simulink library "lib_transmission"  (Simulink 4.1.1)
undefined symbols (not defined in the file or in its folder): fc_map_spd, fc_max_trq, fc_spd_scale, fc_trq_scale, fd_inertia, fd_loss, fd_ratio, gb_inertia, gb_loss_const, gb_loss_input_spd_coeff, gb_loss_input_trq_coeff, gb_loss_output_spd_coeff, gb_loss_output_trq_coeff, gb_map_spd_out, gb_map_trq_in, gb_map_trq_out, gb_ratio, gb_spd_scale, gb_trq_scale, htc_inertia, htc_k_adv, htc_k_adv_coast, htc_max_coast_tr, htc_min_coast_tr, htc_sr, htc_sr_coast, htc_tr, htc_tr_coast, mc_map_spd, mc_max_trq, mc_overtrq_factor, mc_spd_scale, mc_trq_scale, tc_loss, tc_mc_to_fc_ratio, tx_eff_map, tx_map_spd, tx_map_trq, tx_pg_r, tx_pg_s, vc_idle_spd, vc_launch_spd
libraries: lib_transmission x2
(part 2 of 3)

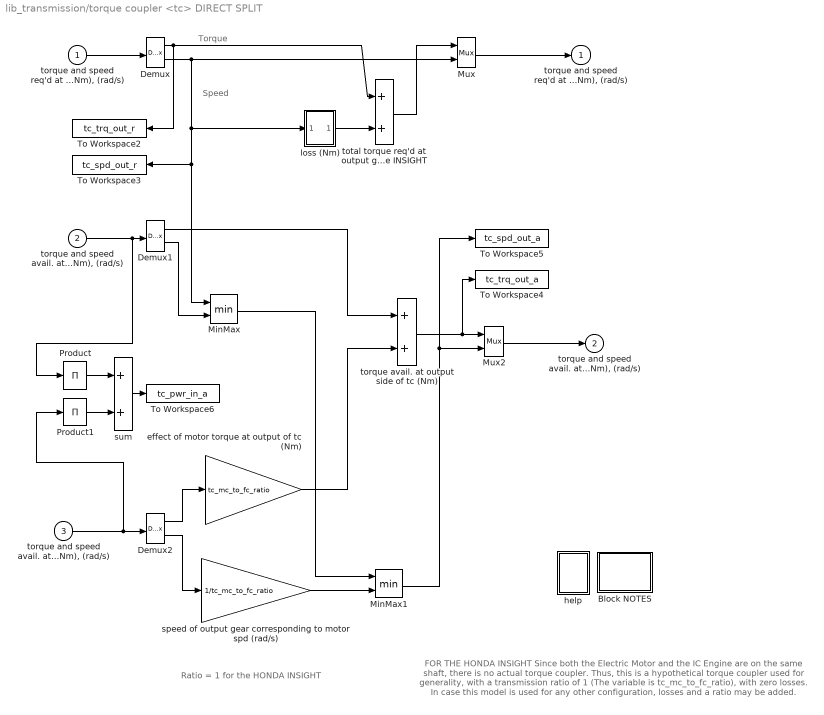
== system lib_transmission/torque coupler <tc> DIRECT SPLIT ==
  note: FOR THE HONDA INSIGHT
      | Since both the Electric Motor and the IC Engine are on the same shaft,
      | there is no actual torque coupler. Thus, this is a hypothetical torque coupler used for
      | generality, with a transmission ratio of 1 (The variable is tc_mc_to_fc_ratio),
      | with zero losses. In case this model is used for any other configuration, losses
      | and a ratio may be added.
  note: Ratio = 1 for the HONDA INSIGHT
  note: Torque
  note: Speed
  "torque and speed req'd at output side of torque coupler (Nm), (rad/s)" : Inport  Port=1  LatchInput=off
  "torque and speed avail. at main input (Nm), (rad/s)" : Inport  Port=2  LatchInput=off
  "torque and speed avail. at motor input to tc (Nm), (rad/s)" : Inport  Port=3  LatchInput=off
  Block NOTES : Subsystem
      settings: RTWFcnNameOpts=Auto  RTWFileNameOpts=Auto
      mask Display: disp('Block\nNOTES')
  Demux : Demux  Outputs=2  BusSelectionMode=off
  Demux1 : Demux  Outputs=2  BusSelectionMode=off
  Demux2 : Demux  Outputs=2  BusSelectionMode=off
  MinMax : MinMax  Function=min  Inputs=2
  MinMax1 : MinMax  Function=min  Inputs=2
  Mux : Mux  Inputs=2
      settings: DisplayOption=none
  Mux2 : Mux  Inputs=2
      settings: DisplayOption=none
  Product : Product  Inputs=1  Multiplication=Element-wise(.*)  SaturateOnIntegerOverflow=on
  Product1 : Product  Inputs=1  Multiplication=Element-wise(.*)  SaturateOnIntegerOverflow=on
  To Workspace2 : ToWorkspace  VariableName=tc_trq_out_r  SampleTime=-1  SaveFormat=Array
  To Workspace3 : ToWorkspace  VariableName=tc_spd_out_r  SampleTime=-1  SaveFormat=Array
  To Workspace4 : ToWorkspace  VariableName=tc_trq_out_a  SampleTime=-1  SaveFormat=Array
  To Workspace5 : ToWorkspace  VariableName=tc_spd_out_a  SampleTime=-1  SaveFormat=Array
  To Workspace6 : ToWorkspace  VariableName=tc_pwr_in_a  SampleTime=-1  SaveFormat=Array
  effect of motor torque at output of tc (Nm) : Gain  Gain=tc_mc_to_fc_ratio  Multiplication=Element-wise(K.*u)  SaturateOnIntegerOverflow=on
  help : Subsystem
      settings: OpenFcn=web(['file:\\\' which('torque_coupler.htm')]);  RTWFcnNameOpts=Auto  RTWFileNameOpts=Auto
      mask Display: image(imread('doc_man.jpg'))
  loss (Nm) : Subsystem
      settings: RTWFcnNameOpts=Auto  RTWFileNameOpts=Auto
  speed of output gear corresponding to motor spd (rad/s) : Gain  Gain=1/tc_mc_to_fc_ratio  Multiplication=Element-wise(K.*u)  SaturateOnIntegerOverflow=on
  "sum " : Sum  Inputs=++  SaturateOnIntegerOverflow=on
  torque avail. at output side of tc (Nm) : Sum  Inputs=++  SaturateOnIntegerOverflow=on
  total torque req'd at output gear (Nm) Loss==0 for the INSIGHT : Sum  Inputs=++  SaturateOnIntegerOverflow=on
  "torque and speed req'd at main input to torque coupler (Nm), (rad/s)" : Outport  Port=1  InitialOutput=0
  "torque and speed avail. at output side of torque coupler (Nm), (rad/s)" : Outport  Port=2  InitialOutput=0
  wires:
  MinMax1/1 -> To Workspace5/1, Mux2/2
  speed of output gear corresponding to motor spd (rad/s)/1 -> MinMax1/2
  Demux2/2 -> speed of output gear corresponding to motor spd (rad/s)/1
  effect of motor torque at output of tc (Nm)/1 -> torque avail. at output side of tc (Nm)/2
  Demux2/1 -> effect of motor torque at output of tc (Nm)/1
  Demux1/2 -> MinMax/2
  "torque and speed req'd at output side of torque coupler (Nm), (rad/s)"/1 -> Demux/1
  Mux/1 -> "torque and speed req'd at main input to torque coupler (Nm), (rad/s)"/1
  "sum "/1 -> To Workspace6/1
  Product/1 -> "sum "/1
  "torque and speed avail. at main input (Nm), (rad/s)"/1 -> Demux1/1, Product/1
  "torque and speed avail. at motor input to tc (Nm), (rad/s)"/1 -> Demux2/1, Product1/1
  Product1/1 -> "sum "/2
  Demux1/1 -> torque avail. at output side of tc (Nm)/1
  MinMax/1 -> MinMax1/1
  Mux2/1 -> "torque and speed avail. at output side of torque coupler (Nm), (rad/s)"/1
  torque avail. at output side of tc (Nm)/1 -> To Workspace4/1, Mux2/1
  Demux/2 -> To Workspace3/1, MinMax/1, loss (Nm)/1(tc output speed (rad/s)), Mux/2
  Demux/1 -> To Workspace2/1, total torque req'd at output gear (Nm) Loss==0 for the INSIGHT/1
  loss (Nm)/1(drag torque (Nm)) -> total torque req'd at output gear (Nm) Loss==0 for the INSIGHT/2
  total torque req'd at output gear (Nm) Loss==0 for the INSIGHT/1 -> Mux/1

== system lib_transmission/CVT gearbox  <gb>/Block NOTES1 ==
  note: This gearbox model includes loss data, rotational inertia, and a gear reduction.
  note: The loss torque is zero when the gears are not turning,
      | and is applied at the input side of the gear reduction.
  note: The inertia torque is the input torque required to accelerate the
      | final drive's inertia as measured on the input side.
  note: Available output torque is estimated assuming that the gearbox efficiency for theavailable input
      | torque andspeed is the same as the gearbox efficiency for the REQUESTED input torque.
  note: This is a good assumption, at least for the VW 4-speed manual transaxle of SAE 820741.
      | In the VW transaxle, efficiency is fairly independent of torque and speed at high torques.

== system lib_transmission/CVT gearbox  <gb>/Pout/Pin, neglecting inertia ==
  note: Pout/Pin, neglecting inertia, is used to estimate the output torque given the
      | input torque in a very simple forward-facing calculation.
  Tin : Inport  Port=1  LatchInput=off
  Tinertia : Inport  Port=2  LatchInput=off
  Tout : Inport  Port=3  LatchInput=off
  gear ratio : Inport  Port=4  LatchInput=off
  Constant : Constant  Orientation=up  Value=eps
  Constant2 : Constant  Orientation=left  Value=0.5
  Pout/Pin (neglecting inertia) : Product  Inputs=*/  Multiplication=Element-wise(.*)  SaturateOnIntegerOverflow=on
  Product : Product  Inputs=2  Multiplication=Element-wise(.*)  SaturateOnIntegerOverflow=on
  Switch : Switch  Threshold=eps
  Tin-Tinertia : Sum  Inputs=+-  SaturateOnIntegerOverflow=on
  make division bombproof : Sum  Inputs=++  SaturateOnIntegerOverflow=on
  Pout/Pin : Outport  Port=1  InitialOutput=0
  wires:
  Switch/1 -> Pout/Pin/1
  Pout/Pin (neglecting inertia)/1 -> Switch/2, Switch/1
  Product/1 -> Pout/Pin (neglecting inertia)/2
  Constant2/1 -> Switch/3
  gear ratio/1 -> Product/1
  make division bombproof/1 -> Product/2
  Tinertia/1 -> Tin-Tinertia/2
  Tout/1 -> Pout/Pin (neglecting inertia)/1
  Tin/1 -> Tin-Tinertia/1
  Tin-Tinertia/1 -> make division bombproof/1
  Constant/1 -> make division bombproof/2

== system lib_transmission/CVT gearbox  <gb>/cvt controller interface ==
  T_gb_out : Inport  Port=1  LatchInput=off
  w_gb_out : Inport  Port=2  LatchInput=off
  eta_gb : Inport  Port=3  LatchInput=off
  gear_ratio : Outport  Port=1  InitialOutput=0
  tag scope: T_gb_out=global, eta_gb=global, w_gb_out=global
  wires:
  T_gb_out/1 -> [T_gb_out]
  w_gb_out/1 -> [w_gb_out]
  eta_gb/1 -> [eta_gb]
  [gear_ratio] -> gear_ratio/1

== system lib_transmission/CVT gearbox  <gb>/effect of inertia (Nm) ==
  note: The inertia torque is the input torque required to accelerate the
      | gearbox's inertia as measured on the input side.
  gb input speed (rad/s) : Inport  Port=1  LatchInput=off
  Gain : Gain  Gain=gb_inertia  Multiplication=Element-wise(K.*u)  SaturateOnIntegerOverflow=on
  d/dt : Derivative
  drag torque (Nm) : Outport  Port=1  InitialOutput=0
  wires:
  Gain/1 -> drag torque (Nm)/1
  gb input speed (rad/s)/1 -> d/dt/1
  d/dt/1 -> Gain/1

== system lib_transmission/CVT gearbox  <gb>/gearbox  efficiency ==
  In1 : Inport  Port=1  LatchInput=off
  Constant : Constant  Value=eps
  Constant1 : Constant  Value=1
  Product : Product  Inputs=*/  Multiplication=Element-wise(.*)  SaturateOnIntegerOverflow=on
  Switch : Switch  Threshold=1
  To Workspace11 : ToWorkspace  VariableName=eta_gb  SampleTime=-1  SaveFormat=Array
  make division bombproof : Sum  Inputs=++  SaturateOnIntegerOverflow=on
  wires:
  Product/1 -> Switch/1
  Constant1/1 -> Product/1
  make division bombproof/1 -> Product/2
  In1/1 -> Switch/3, Switch/2, make division bombproof/1
  Switch/1 -> To Workspace11/1
  Constant/1 -> make division bombproof/2

== system lib_transmission/CVT gearbox  <gb>/gearing (Nm), (rad/s) ==
  "output shaft torque and speed  (Nm), (rad/s)" : Inport  Port=1  LatchInput=off
  gear ratio : Inport  Port=2  LatchInput=off
  Demux : Demux  Outputs=2  BusSelectionMode=off
  Fcn1 : Fcn  Expr=1/u
  Product2 : Product  Inputs=2  Multiplication=Element-wise(.*)  SaturateOnIntegerOverflow=on
  Product3 : Product  Inputs=2  Multiplication=Element-wise(.*)  SaturateOnIntegerOverflow=on
  input shaft torque (Nm) : Outport  Port=1  InitialOutput=0
  input shaft speed (rad/s) : Outport  Port=2  InitialOutput=0
  wires:
  Product3/1 -> input shaft speed (rad/s)/1
  Product2/1 -> input shaft torque (Nm)/1
  Fcn1/1 -> Product2/2
  "output shaft torque and speed  (Nm), (rad/s)"/1 -> Demux/1
  gear ratio/1 -> Fcn1/1, Product3/2
  Demux/1 -> Product2/1
  Demux/2 -> Product3/1

== system lib_transmission/CVT gearbox  <gb>/gearing (Nm), (rad/s)1 ==
  input shaft torque (Nm) : Inport  Port=1  LatchInput=off
  input shaft speed (rad/s) : Inport  Port=2  LatchInput=off
  gear ratio : Inport  Port=3  LatchInput=off
  Fcn1 : Fcn  Expr=1/u
  Product2 : Product  Inputs=2  Multiplication=Element-wise(.*)  SaturateOnIntegerOverflow=on
  Product3 : Product  Inputs=2  Multiplication=Element-wise(.*)  SaturateOnIntegerOverflow=on
  output shaft torque (Nm) : Outport  Port=1  InitialOutput=0
  output shaft speed (rad/s) : Outport  Port=2  InitialOutput=0
  wires:
  input shaft speed (rad/s)/1 -> Product3/2
  input shaft torque (Nm)/1 -> Product2/1
  Product2/1 -> output shaft torque (Nm)/1
  Product3/1 -> output shaft speed (rad/s)/1
  gear ratio/1 -> Fcn1/1, Product2/2
  Fcn1/1 -> Product3/1

== system lib_transmission/CVT gearbox  <gb>/help1 ==

== system lib_transmission/CVT gearbox  <gb>/loss (Nm) ==
  "output torque and speed (Nm), (rad/s)" : Inport  Port=1  LatchInput=off
  pulley ratio : Inport  Port=2  LatchInput=off
  Abs2 : Abs  SaturateOnIntegerOverflow=on
  Demux1 : Demux  Outputs=2  BusSelectionMode=off
  Input Torque: 3-D interpolation : Subsystem
      settings: RTWFcnNameOpts=Auto  RTWFileNameOpts=Auto
  Product3 : Product  Inputs=*/  Multiplication=Element-wise(.*)  SaturateOnIntegerOverflow=on
  Sum2 : Sum  Inputs=-+  SaturateOnIntegerOverflow=on
  loss torque at input shaft (Nm) : Outport  Port=1  InitialOutput=0
  wires:
  Demux1/2 -> Input Torque: 3-D interpolation/2(output speed (rad/s))
  "output torque and speed (Nm), (rad/s)"/1 -> Demux1/1
  pulley ratio/1 -> Input Torque: 3-D interpolation/3(pulley ratio), Product3/2
  Demux1/1 -> Input Torque: 3-D interpolation/1(output torque (N*m)), Product3/1
  Product3/1 -> Sum2/1
  Sum2/1 -> Abs2/1
  Abs2/1 -> loss torque at input shaft (Nm)/1
  Input Torque: 3-D interpolation/1(input torque (Nm)) -> Sum2/2

== system lib_transmission/SubLibraries/3D discrete lookup table ==
  lookup speed (rad/s) : Inport  Port=1  LatchInput=off
  lookup trq (Nm) : Inport  Port=2  LatchInput=off
  "gear_number  (e.g., 1, 2, 3)" : Inport  Port=3  LatchInput=off
  Mux : Mux  Inputs=3
  Saturation : Saturate  UpperLimit=max(tx_map_spd)  LowerLimit=min(tx_map_spd)  LinearizeAsGain=on
  Saturation1 : Saturate  UpperLimit=max(tx_map_trq)  LowerLimit=min(tx_map_trq)  LinearizeAsGain=on
  Saturation2 : Saturate  UpperLimit=size(tx_eff_map,3)  LowerLimit=1  LinearizeAsGain=on
  interp2d : MATLABFcn  MATLABFcn=interp2(tx_map_trq, tx_map_spd, tx_eff_map(:,:,u(3)),u(2),u(1))  OutputDimensions=1  OutputSignalType=real  Output1D=on
  tx_eff : Outport  Port=1
  wires:
  Mux/1 -> interp2d/1
  interp2d/1 -> tx_eff/1
  lookup speed (rad/s)/1 -> Saturation/1
  Saturation/1 -> Mux/1
  lookup trq (Nm)/1 -> Saturation1/1
  Saturation1/1 -> Mux/2
  "gear_number  (e.g., 1, 2, 3)"/1 -> Saturation2/1
  Saturation2/1 -> Mux/3

== system lib_transmission/SubLibraries/3D discrete lookup table (sfun) ==
  lookup speed (rad/s) : Inport  Port=1  LatchInput=off
  lookup trq (Nm) : Inport  Port=2  LatchInput=off
  "gear_number  (e.g., 1, 2, 3)" : Inport  Port=3  LatchInput=off
  Mux : Mux  Inputs=3
  Saturation : Saturate  UpperLimit=max(tx_map_spd)  LowerLimit=min(tx_map_spd)  LinearizeAsGain=on
  Saturation1 : Saturate  UpperLimit=max(tx_map_trq)  LowerLimit=min(tx_map_trq)  LinearizeAsGain=on
  Saturation2 : Saturate  UpperLimit=size(tx_eff_map,3)  LowerLimit=1  LinearizeAsGain=on
  discrete interp2d : S-Function  FunctionName=sfun_discreteLookup3d  Parameters=tx_map_trq, tx_map_spd, tx_eff_map  PortCounts=[]  SFunctionModules=''
  tx_eff : Outport  Port=1
  wires:
  Saturation2/1 -> Mux/3
  "gear_number  (e.g., 1, 2, 3)"/1 -> Saturation2/1
  Saturation1/1 -> Mux/2
  lookup trq (Nm)/1 -> Saturation1/1
  Saturation/1 -> Mux/1
  lookup speed (rad/s)/1 -> Saturation/1
  Mux/1 -> discrete interp2d/1
  discrete interp2d/1 -> tx_eff/1

== system lib_transmission/SubLibraries/gear determination (e.g., 1st gear, 2nd, etc.) ==
  in_1 : Inport  Port=1  LatchInput=off
  Look-Up Table : Lookup  InputValues=fliplr([gb_ratio(1)+0.00001,gb_ratio(2:end)])  OutputValues=fliplr( [1:length(gb_ratio)] )
  Rounding Function : Rounding  Operator=round
  index of lower bounding map : Outport  Port=1  InitialOutput=0
  wires:
  in_1/1 -> Look-Up Table/1
  Look-Up Table/1 -> Rounding Function/1
  Rounding Function/1 -> index of lower bounding map/1

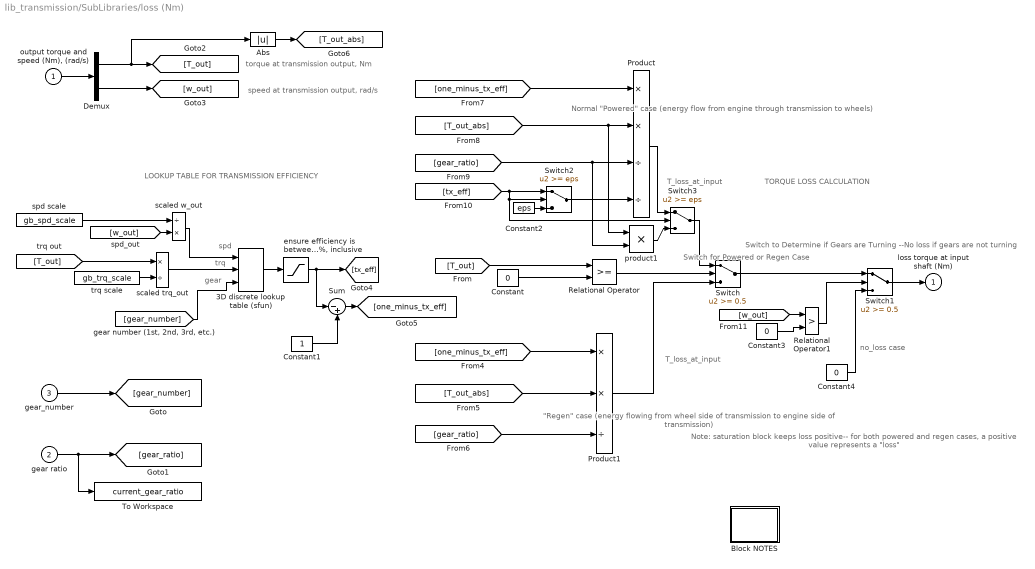
== system lib_transmission/SubLibraries/loss (Nm) ==
  note: LOOKUP TABLE FOR TRANSMISSION EFFICIENCY
  note: T_loss_at_input
  note: "Regen" case
      | (energy flowing from
      | wheel side of transmission
      | to engine side of transmission)
  note: T_loss_at_input
  note: Normal "Powered" case
      | (energy flow from engine
      | through transmission to wheels)
  note: Switch to Determine
      | if Gears are Turning
      | --No loss if gears
      | are not turning
  note: Switch for Powered
      |  or Regen Case
  note: Note: saturation block keeps
      | loss positive-- for both powered
      | and regen cases, a
      | positive value represents a "loss"
  note: no_loss case
  note: speed at transmission output, rad/s
  note: torque at transmission output, Nm
  note: spd
  note: trq
  note: gear
  note: TORQUE LOSS CALCULATION
  "output torque and speed (Nm), (rad/s)" : Inport  Port=1  LatchInput=off
  gear ratio : Inport  Port=2  LatchInput=off
  gear_number : Inport  Port=3  LatchInput=off
  3D discrete lookup table (sfun) : lib_transmission/SubLibraries/3D discrete lookup table (sfun)  tx_map_spd=tx_map_spd  tx_map_trq=tx_map_trq  tx_eff_map=tx_eff_map
  Abs : Abs  SaturateOnIntegerOverflow=on
  Block NOTES : Subsystem
      settings: RTWFcnNameOpts=Auto  RTWFileNameOpts=Auto
      mask Display: disp('Block\nNOTES')
  Constant : Constant  Value=0
  Constant1 : Constant  Value=1
  Constant2 : Constant  Value=eps
  Constant3 : Constant  Value=0
  Constant4 : Constant  Value=0
  Demux : Demux  Outputs=2  BusSelectionMode=off
  Product : Product  Inputs=**//  Multiplication=Element-wise(.*)  SaturateOnIntegerOverflow=on
  Product1 : Product  Inputs=**/  Multiplication=Element-wise(.*)  SaturateOnIntegerOverflow=on
  Relational Operator : RelationalOperator  Operator=>=
  Relational Operator1 : RelationalOperator  Operator=>
  Sum : Sum  Inputs=|-+  SaturateOnIntegerOverflow=on
  Switch : Switch  Threshold=0.5
  Switch1 : Switch  Threshold=0.5
  Switch2 : Switch  Threshold=eps
  Switch3 : Switch  Threshold=eps
  To Workspace : ToWorkspace  VariableName=current_gear_ratio  SampleTime=-1  SaveFormat=Array
      settings: MaxDataPoints=1
  "ensure efficiency is between  0% and 100%, inclusive" : Saturate  UpperLimit=1  LowerLimit=0  LinearizeAsGain=on
  product1 : Product  Inputs=2  Multiplication=Element-wise(.*)  SaturateOnIntegerOverflow=on
  scaled trq_out : Product  Inputs=*/  Multiplication=Element-wise(.*)  SaturateOnIntegerOverflow=on
  scaled w_out : Product  Inputs=/*  Multiplication=Element-wise(.*)  SaturateOnIntegerOverflow=on
  spd scale : Constant  Value=gb_spd_scale
  trq scale : Constant  Value=gb_trq_scale
  loss torque at input shaft (Nm) : Outport  Port=1  InitialOutput=0
  wires:
  "output torque and speed (Nm), (rad/s)"/1 -> Demux/1
  Demux/2 -> [w_out]
  [gear_number] -> 3D discrete lookup table (sfun)/3
  Relational Operator/1 -> Switch/2
  Constant/1 -> Relational Operator/2
  [T_out] -> Relational Operator/1
  Product1/1 -> Switch/3
  [one_minus_tx_eff] -> Product1/1
  [gear_ratio] -> Product1/3
  [T_out_abs] -> Product1/2
  [one_minus_tx_eff] -> Product/1
  [T_out_abs] -> Product/2, product1/1
  [gear_ratio] -> Product/3, product1/2
  Switch1/1 -> loss torque at input shaft (Nm)/1
  Constant4/1 -> Switch1/3
  [w_out] -> Relational Operator1/1
  Constant3/1 -> Relational Operator1/2
  Relational Operator1/1 -> Switch1/2
  Demux/1 -> [T_out], Abs/1
  Abs/1 -> [T_out_abs]
  Switch/1 -> Switch1/1
  3D discrete lookup table (sfun)/1 -> "ensure efficiency is between  0% and 100%, inclusive"/1
  "ensure efficiency is between  0% and 100%, inclusive"/1 -> [tx_eff], Sum/1
  scaled w_out/1 -> 3D discrete lookup table (sfun)/1
  [T_out] -> scaled trq_out/1
  scaled trq_out/1 -> 3D discrete lookup table (sfun)/2
  trq scale/1 -> scaled trq_out/2
  Constant1/1 -> Sum/2
  Sum/1 -> [one_minus_tx_eff]
  [w_out] -> scaled w_out/2
  spd scale/1 -> scaled w_out/1
  gear ratio/1 -> [gear_ratio], To Workspace/1
  gear_number/1 -> [gear_number]
  Switch2/1 -> Product/4
  [tx_eff] -> Switch2/1, Switch2/2, Switch3/2
  Constant2/1 -> Switch2/3
  Switch3/1 -> Switch/1
  Product/1 -> Switch3/1
  product1/1 -> Switch3/3

== system lib_transmission/SubLibraries/loss (Nm) old methodology ==
  note: Loss torque applied at input side is a function of
      |  output speed, output torque, and gear number.
      | There is no loss if the gears are not turning.
  "output torque and speed (Nm), (rad/s)" : Inport  Port=1  LatchInput=off
  gear ratio : Inport  Port=2  LatchInput=off
  Abs : Abs  SaturateOnIntegerOverflow=on
  Block NOTES : Subsystem
      settings: RTWFcnNameOpts=Auto  RTWFileNameOpts=Auto
      mask Display: disp('Block\nNOTES')
  Constant : Constant  Orientation=up  Value=eps
  Constant1 : Constant  Value=gb_loss_input_spd_coeff/gb_spd_scale
  Constant2 : Constant  Value=gb_loss_input_trq_coeff/gb_trq_scale
  Constant3 : Constant  Value=gb_loss_output_spd_coeff/gb_spd_scale
  Constant4 : Constant  Value=gb_loss_output_trq_coeff/gb_trq_scale
  Constant5 : Constant  Orientation=up  Value=gb_loss_const
  Constant6 : Constant  Value=gb_loss_output_pwr_coeff/gb_spd_scale/gb_trq_scale
  Constant7 : Constant  Orientation=up  Value=0
  Demux : Demux  Outputs=2  BusSelectionMode=off
  Product : Product  Inputs=2  Multiplication=Element-wise(.*)  SaturateOnIntegerOverflow=on
  Product1 : Product  Inputs=/*  Multiplication=Element-wise(.*)  SaturateOnIntegerOverflow=on
  Product2 : Product  Inputs=2  Multiplication=Element-wise(.*)  SaturateOnIntegerOverflow=on
  Product3 : Product  Inputs=2  Multiplication=Element-wise(.*)  SaturateOnIntegerOverflow=on
  Product4 : Product  Inputs=3  Multiplication=Element-wise(.*)  SaturateOnIntegerOverflow=on
  Relational Operator : RelationalOperator  Operator=>
  Saturation : Saturate  UpperLimit=inf  LowerLimit=0  LinearizeAsGain=on
  Sum : Sum  Inputs=++  SaturateOnIntegerOverflow=on
  Sum1 : Sum  Inputs=++  SaturateOnIntegerOverflow=on
  Sum2 : Sum  Inputs=++++  SaturateOnIntegerOverflow=on
  Sum3 : Sum  Orientation=up  Inputs=++  SaturateOnIntegerOverflow=on
  Switch : Switch  Threshold=eps
  loss torque : Product  Inputs=*//  Multiplication=Element-wise(.*)  SaturateOnIntegerOverflow=on
  loss torque at input shaft (Nm) : Outport  Port=1  InitialOutput=0
  wires:
  Abs/1 -> Product2/1, Product4/1
  Demux/1 -> Abs/1
  Relational Operator/1 -> Switch/2
  Constant/1 -> Relational Operator/2, Sum3/2
  Constant7/1 -> Switch/3
  Product3/1 -> Sum2/3
  Product2/1 -> Sum2/1
  "output torque and speed (Nm), (rad/s)"/1 -> Demux/1
  Constant1/1 -> Product/2
  Product/1 -> Sum1/2
  Sum/1 -> Product2/2
  Sum1/1 -> Product3/2
  Constant5/1 -> Sum2/4
  gear ratio/1 -> Product1/1, Product/1, loss torque/3
  Constant2/1 -> Product1/2
  Product1/1 -> Sum/2
  Constant4/1 -> Sum/1
  Constant3/1 -> Sum1/1
  Constant6/1 -> Product4/2
  Product4/1 -> Sum2/2
  Switch/1 -> loss torque at input shaft (Nm)/1
  Sum2/1 -> loss torque/1
  Demux/2 -> Product3/1, Product4/3, Relational Operator/1, Sum3/1
  loss torque/1 -> Saturation/1
  Saturation/1 -> Switch/1
  Sum3/1 -> loss torque/2

== system lib_transmission/SubLibraries/notes on  3D discrete lookup table ==
  note: performs a "2D" lookup
      | for the specified
      | z height of the 3D lookup matrix
      | (i.e., no interpolation on z, only discrete)
  note: created 5 July 2001 mpo
      | Revision history:
      | ...
  note: 3 inputs:
      | (1) X lookup
      | (2) Y lookup
      | (3) discrete Z value (integer)
      |
      | 1 output:
      | (1) looked up value
  note: 3 masked inputs:
      | (1) array of X values in table
      | (2) array of Y values in table
      | (3) 3D lookup table (i.e., 2D tables for several Z values)

== system lib_transmission/SubLibraries/notes on  loss (Nm) ==
  note: 4 masked inputs:
      | (1) map of efficiencies by spd and trq and gear number (discrete)
      | (2) array of trq values in efficiency map lookup table
      | (3) array of spd values in efficiency map lookup table
      | (4) the ratios in the gear box
  note: 2 inputs:
      | (1) trq and spd at output (wheel side)
      | of Transmission (muxxed)
      | (2) current gear ratio
      |
      | 1 output:
      | (1) trq loss at input (engine side) of
      | transmission
  note: created 5 July 2001 mpo
      | Revision history:
      | ...
  note: Calculates the torque loss due to
      | transmission inefficiencies
      | (torque lost at input to transmission)
  note: note: tx_map_spd and tx_map_trq
      |  are output (wheelside) values
  note: data needs:
      | tx_map_spd
      | tx_map_trq
      | tx_eff_map
      | gb_ratio

== system lib_transmission/clutch <cl>/help ==

== system lib_transmission/clutch <cl> for par S/A/help ==

== system lib_transmission/clutch par CVT <cl>/help ==

== system lib_transmission/final drive <fd>/Block NOTES ==
  note: This final drive model includes loss data, rotational inertia, and a gear reduction.
  note: The loss torque is zero when the gears are not turning,
      | and is applied at the input side of the gear reduction.
  note: The inertia torque is the input torque required to accelerate the
      | final drive's inertia as measured on the input side.

== system lib_transmission/final drive <fd>/effect of inertia (Nm) ==
  note: The inertia torque is the input torque required to accelerate the
      | final drive's inertia as measured on the input side.
  fd input speed (rad/s) : Inport  Port=1  LatchInput=off
  Gain : Gain  Gain=fd_inertia  Multiplication=Element-wise(K.*u)  SaturateOnIntegerOverflow=on
  d/dt : Derivative
  drag torque (Nm) : Outport  Port=1  InitialOutput=0
  wires:
  Gain/1 -> drag torque (Nm)/1
  d/dt/1 -> Gain/1
  fd input speed (rad/s)/1 -> d/dt/1

== system lib_transmission/final drive <fd>/help ==

== system lib_transmission/final drive <fd>/loss (Nm) ==
  note: The loss torque is zero when the gears are not turning,
      | and is applied at the input side of the gear reduction.
  fd output speed (rad/s) : Inport  Port=1  LatchInput=off
  Constant : Constant  Orientation=up  Value=0
  Switch : Switch  Threshold=eps
  final drive loss torque (Nm) : Constant  Value=fd_loss
  drag torque (Nm) : Outport  Port=1  InitialOutput=0
  wires:
  final drive loss torque (Nm)/1 -> Switch/1
  Switch/1 -> drag torque (Nm)/1
  fd output speed (rad/s)/1 -> Switch/2
  Constant/1 -> Switch/3

== system lib_transmission/gearbox <gb>/Block NOTES ==
  note: This gearbox model includes loss data, rotational inertia, and a gear reduction.
  note: The loss torque is zero when the gears are not turning,
      | and is applied at the input side of the gear reduction.
  note: The inertia torque is the input torque required to accelerate the
      | final drive's inertia as measured on the input side.
  note: Available output torque is estimated assuming that the gearbox efficiency for theavailable input
      | torque andspeed is the same as the gearbox efficiency for the REQUESTED input torque.
  note: This is a good assumption, at least for the VW 4-speed manual transaxle of SAE 820741.
      | In the VW transaxle, efficiency is fairly independent of torque and speed at high torques.

== system lib_transmission/gearbox <gb>/Pout/Pin, neglecting inertia ==
  note: Pout/Pin, neglecting inertia, is used to estimate the output torque given the
      | input torque in a very simple forward-facing calculation.
  Tin : Inport  Port=1  LatchInput=off
  Tinertia : Inport  Port=2  LatchInput=off
  Tout : Inport  Port=3  LatchInput=off
  gear ratio : Inport  Port=4  LatchInput=off
  Constant1 : Constant  Orientation=up  Value=0
  Pout/Pin (neglecting inertia) : Subsystem
      settings: RTWFcnNameOpts=Auto  RTWFileNameOpts=Auto
      mask Display: disp('/')
  Product : Product  Inputs=2  Multiplication=Element-wise(.*)  SaturateOnIntegerOverflow=on
  Relational Operator : RelationalOperator  Operator=~=
  Saturation : Saturate  UpperLimit=inf  LowerLimit=0  LinearizeAsGain=on
  Switch : Switch  Threshold=eps
  Tin-Tinertia : Sum  Inputs=+-  SaturateOnIntegerOverflow=on
  make division bombproof : Subsystem
      settings: RTWFcnNameOpts=Auto  RTWFileNameOpts=Auto
  Pout/Pin : Outport  Port=1  InitialOutput=0
  wires:
  Constant1/1 -> Switch/3, Relational Operator/2
  make division bombproof/1(Out1) -> Product/2
  Tinertia/1 -> Tin-Tinertia/2
  Tin/1 -> Tin-Tinertia/1
  Pout/Pin (neglecting inertia)/1(out_1) -> Switch/1
  Relational Operator/1 -> Switch/2
  Switch/1 -> Saturation/1
  Saturation/1 -> Pout/Pin/1
  Tin-Tinertia/1 -> make division bombproof/1(Tin-Tinertia), Relational Operator/1
  Tout/1 -> Pout/Pin (neglecting inertia)/1(in_1)
  Product/1 -> Pout/Pin (neglecting inertia)/2(in_2)
  gear ratio/1 -> Product/1

== system lib_transmission/gearbox <gb>/effect of inertia (Nm) ==
  note: The inertia torque is the input torque required to accelerate the
      | gearbox's inertia as measured on the input side.
  gb input speed (rad/s) : Inport  Port=1  LatchInput=off
  Gain : Gain  Gain=gb_inertia  Multiplication=Element-wise(K.*u)  SaturateOnIntegerOverflow=on
  d/dt : Derivative
  drag torque (Nm) : Outport  Port=1  InitialOutput=0
  wires:
  Gain/1 -> drag torque (Nm)/1
  d/dt/1 -> Gain/1
  gb input speed (rad/s)/1 -> d/dt/1

== system lib_transmission/gearbox <gb>/gearbox controller interface ==
  T_gb_out : Inport  Port=1  LatchInput=off
  w_gb_out : Inport  Port=2  LatchInput=off
  eta_gb : Inport  Port=3  LatchInput=off
  gear_ratio : Outport  Port=1  InitialOutput=0
  shifting : Outport  Port=2  InitialOutput=0
  tag scope: T_gb_out=global, eta_gb=global, w_gb_out=global
  wires:
  [gear_ratio] -> gear_ratio/1
  eta_gb/1 -> [eta_gb]
  w_gb_out/1 -> [w_gb_out]
  T_gb_out/1 -> [T_gb_out]
  [shifting] -> shifting/1

== system lib_transmission/gearbox <gb>/gearing (Nm), (rad/s) ==
  "output shaft torque and speed  (Nm), (rad/s)" : Inport  Port=1  LatchInput=off
  gear ratio : Inport  Port=2  LatchInput=off
  Demux : Demux  Outputs=2  BusSelectionMode=off
  Fcn1 : Fcn  Expr=1/u
  Product2 : Product  Inputs=2  Multiplication=Element-wise(.*)  SaturateOnIntegerOverflow=on
  Product3 : Product  Inputs=2  Multiplication=Element-wise(.*)  SaturateOnIntegerOverflow=on
  input shaft torque (Nm) : Outport  Port=1  InitialOutput=0
  input shaft speed (rad/s) : Outport  Port=2  InitialOutput=0
  wires:
  Product3/1 -> input shaft speed (rad/s)/1
  Product2/1 -> input shaft torque (Nm)/1
  Fcn1/1 -> Product2/2
  "output shaft torque and speed  (Nm), (rad/s)"/1 -> Demux/1
  gear ratio/1 -> Fcn1/1, Product3/2
  Demux/1 -> Product2/1
  Demux/2 -> Product3/1

== system lib_transmission/gearbox <gb>/gearing (Nm), (rad/s)1 ==
  input shaft torque (Nm) : Inport  Port=1  LatchInput=off
  input shaft speed (rad/s) : Inport  Port=2  LatchInput=off
  gear ratio : Inport  Port=3  LatchInput=off
  Fcn1 : Fcn  Expr=1/u
  Product2 : Product  Inputs=2  Multiplication=Element-wise(.*)  SaturateOnIntegerOverflow=on
  Product3 : Product  Inputs=2  Multiplication=Element-wise(.*)  SaturateOnIntegerOverflow=on
  output shaft torque (Nm) : Outport  Port=1  InitialOutput=0
  output shaft speed (rad/s) : Outport  Port=2  InitialOutput=0
  wires:
  Fcn1/1 -> Product3/1
  gear ratio/1 -> Product2/2, Fcn1/1
  Product3/1 -> output shaft speed (rad/s)/1
  Product2/1 -> output shaft torque (Nm)/1
  input shaft torque (Nm)/1 -> Product2/1
  input shaft speed (rad/s)/1 -> Product3/2

== system lib_transmission/gearbox <gb>/help ==

== system lib_transmission/hydraulic torque converter <htc>/Block NOTES ==
  note: This block predicts the relative speed of the HTC input (pump) and output
      | (turbine).  Torque converter lockup is modeled.
      |
      | 1/24/00:tm updated gear_ratio flag to shifting flag

== system lib_transmission/hydraulic torque converter <htc>/SR ==
  T,w req out : Inport  Port=1  LatchInput=off
  w in : Inport  Port=2  LatchInput=off
  >0 : Saturate  UpperLimit=inf  LowerLimit=eps  LinearizeAsGain=on
  Constant : Constant  Orientation=left  Value=0
  Constant1 : Constant  Value=vc_idle_spd+eps
  Constant3 : Constant  Value=1
  K_adv : Subsystem
      settings: RTWFcnNameOpts=Auto  RTWFileNameOpts=Auto
  K_adv_coast : Subsystem
      settings: RTWFcnNameOpts=Auto  RTWFileNameOpts=Auto
  Logical Operator : Logic  Operator=NOT  Inputs=1
  Logical Operator1 : Logic  Operator=NOT  Inputs=1
  MinMax : MinMax  Function=min  Inputs=2
  Relational Operator : RelationalOperator  Operator=>=
  SR Look-Up Table SR=wout/win : Lookup  InputValues=htc_k_adv  OutputValues=htc_sr
  SR Look-Up Table SR=wout/win coast : Lookup  InputValues=fliplr(htc_k_adv_coast)  OutputValues=fliplr(htc_sr_coast)
  SRmax= wout/win,min : Product  Inputs=*/  Multiplication=Element-wise(.*)  SaturateOnIntegerOverflow=on
  T : Selector  InputType=Vector  ElementSrc=Internal  Elements=1  RowSrc=Internal  Rows=1  ColumnSrc=Internal  Columns=1  InputPortWidth=2
  To Workspace1 : ToWorkspace  VariableName=htc_locked  SampleTime=-1  SaveFormat=Array
  To Workspace3 : ToWorkspace  VariableName=htc_coasting  SampleTime=-1  SaveFormat=Array
  if coasting : Switch  Threshold=eps
  "locked up, then SR=1" : Switch  Threshold=eps
  min,max : Saturate  UpperLimit=inf  LowerLimit=1  LinearizeAsGain=on
  shifting SR : Subsystem
      settings: RTWFcnNameOpts=Auto  RTWFileNameOpts=Auto
  wout,req : Selector  InputType=Vector  ElementSrc=Internal  Elements=2  RowSrc=Internal  Rows=1  ColumnSrc=Internal  Columns=1  InputPortWidth=2
  SR : Outport  Port=1  InitialOutput=0
  coasting : Outport  Port=2  InitialOutput=0
  wires:
  K_adv/1(K_adv) -> SR Look-Up Table SR=wout/win/1
  Logical Operator1/1 -> coasting/1, To Workspace3/1
  >0/1 -> SR/1
  if coasting/1 -> >0/1
  K_adv_coast/1(K_adv_coast) -> SR Look-Up Table SR=wout/win coast/1
  MinMax/1 -> if coasting/3
  min,max/1 -> MinMax/1
  wout,req/1 -> SRmax= wout/win,min/1
  Constant1/1 -> SRmax= wout/win,min/2
  SRmax= wout/win,min/1 -> MinMax/2
  shifting SR/1(SR limited) -> if coasting/1
  "locked up, then SR=1"/1 -> shifting SR/3(SR)
  w in/1 -> shifting SR/2(w in)
  SR Look-Up Table SR=wout/win/1 -> "locked up, then SR=1"/1
  Constant3/1 -> "locked up, then SR=1"/3
  Logical Operator/1 -> "locked up, then SR=1"/2
  Relational Operator/1 -> Logical Operator1/1, if coasting/2
  T/1 -> Relational Operator/1
  Constant/1 -> Relational Operator/2
  SR Look-Up Table SR=wout/win coast/1 -> min,max/1
  T,w req out/1 -> shifting SR/1(T,w req out), K_adv/1("Req'd output trq and spd (Nm), (rad/s)"), wout,req/1, K_adv_coast/1("Req'd output trq and spd (Nm), (rad/s)"), T/1
  [locked_up] -> Logical Operator/1, To Workspace1/1

== system lib_transmission/hydraulic torque converter <htc>/T, shifting ==
  TR : Inport  Port=1  LatchInput=off
  Req'd  input trq : Inport  Port=2  LatchInput=off
  Req'd output trq : Inport  Port=3  LatchInput=off
  htc_spd_in_a : Inport  Port=4  LatchInput=off
  SR : Inport  Port=5  LatchInput=off
  Memory : Memory  X0=0  InheritSampleTime=off
      settings: RTWStateStorageClass=Auto
  Memory1 : Memory  X0=0  InheritSampleTime=off
      settings: RTWStateStorageClass=Auto
  MinMax : MinMax  Function=min  Inputs=2
  TR Look-Up Table TR=Tout/Tin : Lookup  InputValues=htc_sr  OutputValues=htc_tr
  T_max : Subsystem
      settings: RTWFcnNameOpts=Auto  RTWFileNameOpts=Auto
  Tin*TR= Tout,req : Product  Inputs=2  Multiplication=Element-wise(.*)  SaturateOnIntegerOverflow=on
  engine speed estimator : Subsystem
      settings: RTWFcnNameOpts=Auto  RTWFileNameOpts=Auto
  "shifting, override zero Trequest" : Switch  Threshold=eps
  T req : Outport  Port=1
  wires:
  Tin*TR= Tout,req/1 -> Memory/1
  TR/1 -> Tin*TR= Tout,req/2
  Req'd  input trq/1 -> Tin*TR= Tout,req/1
  Memory/1 -> "shifting, override zero Trequest"/1
  T_max/1(T_max max gain from htc) -> MinMax/2
  "shifting, override zero Trequest"/1 -> MinMax/1
  TR Look-Up Table TR=Tout/Tin/1 -> T_max/2(TR)
  MinMax/1 -> T req/1
  engine speed estimator/1(Out1) -> T_max/1(w_APU)
  Memory1/1 -> TR Look-Up Table TR=Tout/Tin/1
  SR/1 -> Memory1/1
  htc_spd_in_a/1 -> engine speed estimator/1(htc_spd_in_a)
  Req'd output trq/1 -> "shifting, override zero Trequest"/3
  [shifting] -> "shifting, override zero Trequest"/2

== system lib_transmission/hydraulic torque converter <htc>/TR ==
  SR : Inport  Port=1  LatchInput=off
  coasting : Inport  Port=2  LatchInput=off
  1/SR*TR  for coast : Fcn  Expr=1/u
  Constant3 : Constant  Value=1
  Logical Operator : Logic  Operator=NOT  Inputs=1
  Logical Operator1 : Logic  Operator=NOT  Inputs=1
  TR Look-Up Table TR=Tout/Tin : Lookup  InputValues=htc_sr  OutputValues=htc_tr
  TR Look-Up Table TR=Tout/Tin coast : Lookup  InputValues=htc_sr_coast  OutputValues=htc_tr_coast
  To Workspace11 : ToWorkspace  VariableName=htc_efficiency  SampleTime=-1  SaveFormat=Array
  effic=SR*TR : Product  Inputs=**  Multiplication=Element-wise(.*)  SaturateOnIntegerOverflow=on
  if coasting : Switch  Threshold=eps
  if coasting1 : Switch  Threshold=eps
  "locked up, then TR=1" : Switch  Threshold=eps
  min,max : Saturate  UpperLimit=htc_max_coast_tr  LowerLimit=htc_min_coast_tr  LinearizeAsGain=on
  TR : Outport  Port=1  InitialOutput=0
  wires:
  if coasting1/1 -> To Workspace11/1
  1/SR*TR  for coast/1 -> if coasting1/3
  effic=SR*TR/1 -> 1/SR*TR  for coast/1, if coasting1/1
  Logical Operator1/1 -> if coasting1/2, if coasting/2
  if coasting/1 -> effic=SR*TR/2, TR/1
  coasting/1 -> Logical Operator1/1
  SR/1 -> effic=SR*TR/1, TR Look-Up Table TR=Tout/Tin/1, TR Look-Up Table TR=Tout/Tin coast/1
  min,max/1 -> if coasting/3
  TR Look-Up Table TR=Tout/Tin coast/1 -> min,max/1
  "locked up, then TR=1"/1 -> if coasting/1
  Logical Operator/1 -> "locked up, then TR=1"/2
  [locked_up] -> Logical Operator/1
  Constant3/1 -> "locked up, then TR=1"/3
  TR Look-Up Table TR=Tout/Tin/1 -> "locked up, then TR=1"/1

== system lib_transmission/hydraulic torque converter <htc>/effect of inertia (Nm) ==
  note: This block computes the torque required to overcome the inertia of the
      | turbine (plus 1/2 fluid in htc).
  turbine/output speed (rad/s) : Inport  Port=1  LatchInput=off
  Constant : Constant  Value=htc_inertia
  Product : Product  Inputs=2  Multiplication=Element-wise(.*)  SaturateOnIntegerOverflow=on
  d/dt : Derivative
  inertia torque (Nm) : Outport  Port=1  InitialOutput=0
  wires:
  Product/1 -> inertia torque (Nm)/1
  Constant/1 -> Product/2
  turbine/output speed (rad/s)/1 -> d/dt/1
  d/dt/1 -> Product/1

== system lib_transmission/hydraulic torque converter for  parallel hybrid <htc>/Block NOTES ==
  note: This block predicts the relative speed of the HTC input (pump) and output
      | (turbine).  Torque converter lockup is modeled.

== system lib_transmission/hydraulic torque converter for  parallel hybrid <htc>/SR ==
  T,w req out : Inport  Port=1  LatchInput=off
  w in : Inport  Port=2  LatchInput=off
  >0 : Saturate  UpperLimit=inf  LowerLimit=eps  LinearizeAsGain=on
  Constant : Constant  Orientation=left  Value=0
  Constant1 : Constant  Value=vc_idle_spd+eps
  Constant3 : Constant  Value=1
  K_adv : Subsystem
      settings: RTWFcnNameOpts=Auto  RTWFileNameOpts=Auto
  K_adv_coast : Subsystem
      settings: RTWFcnNameOpts=Auto  RTWFileNameOpts=Auto
  Logical Operator : Logic  Operator=NOT  Inputs=1
  Logical Operator1 : Logic  Operator=NOT  Inputs=1
  MinMax : MinMax  Function=min  Inputs=2
  Relational Operator : RelationalOperator  Operator=>=
  SR Look-Up Table SR=wout/win : Lookup  InputValues=htc_k_adv  OutputValues=htc_sr
  SR Look-Up Table SR=wout/win coast : Lookup  InputValues=fliplr(htc_k_adv_coast)  OutputValues=fliplr(htc_sr_coast)
  SRmax= wout/win,min : Product  Inputs=*/  Multiplication=Element-wise(.*)  SaturateOnIntegerOverflow=on
  T : Selector  InputType=Vector  ElementSrc=Internal  Elements=1  RowSrc=Internal  Rows=1  ColumnSrc=Internal  Columns=1  InputPortWidth=2
  To Workspace1 : ToWorkspace  VariableName=htc_locked  SampleTime=-1  SaveFormat=Array
  To Workspace3 : ToWorkspace  VariableName=htc_coasting  SampleTime=-1  SaveFormat=Array
  if coasting : Switch  Threshold=eps
  "locked up, then SR=1" : Switch  Threshold=eps
  min,max : Saturate  UpperLimit=inf  LowerLimit=1  LinearizeAsGain=on
  shifting SR : Subsystem
      settings: RTWFcnNameOpts=Auto  RTWFileNameOpts=Auto
  wout,req : Selector  InputType=Vector  ElementSrc=Internal  Elements=2  RowSrc=Internal  Rows=1  ColumnSrc=Internal  Columns=1  InputPortWidth=2
  SR : Outport  Port=1  InitialOutput=0
  coasting : Outport  Port=2  InitialOutput=0
  wires:
  K_adv/1(K_adv) -> SR Look-Up Table SR=wout/win/1
  Logical Operator1/1 -> coasting/1, To Workspace3/1
  >0/1 -> SR/1
  if coasting/1 -> >0/1
  K_adv_coast/1(K_adv_coast) -> SR Look-Up Table SR=wout/win coast/1
  MinMax/1 -> if coasting/3
  min,max/1 -> MinMax/1
  wout,req/1 -> SRmax= wout/win,min/1
  Constant1/1 -> SRmax= wout/win,min/2
  SRmax= wout/win,min/1 -> MinMax/2
  shifting SR/1(SR limited) -> if coasting/1
  "locked up, then SR=1"/1 -> shifting SR/3(SR)
  w in/1 -> shifting SR/2(w in)
  SR Look-Up Table SR=wout/win/1 -> "locked up, then SR=1"/1
  Constant3/1 -> "locked up, then SR=1"/3
  Logical Operator/1 -> "locked up, then SR=1"/2
  T/1 -> Relational Operator/1
  Constant/1 -> Relational Operator/2
  SR Look-Up Table SR=wout/win coast/1 -> min,max/1
  T,w req out/1 -> shifting SR/1(T,w req out), K_adv/1("Req'd output trq and spd (Nm), (rad/s)"), wout,req/1, K_adv_coast/1("Req'd output trq and spd (Nm), (rad/s)"), T/1
  [locked_up] -> Logical Operator/1, To Workspace1/1
  Relational Operator/1 -> Logical Operator1/1, if coasting/2

== system lib_transmission/hydraulic torque converter for  parallel hybrid <htc>/T, shifting ==
  TR : Inport  Port=1  LatchInput=off
  Req'd  input trq : Inport  Port=2  LatchInput=off
  Req'd output trq : Inport  Port=3  LatchInput=off
  htc_spd_in_a : Inport  Port=4  LatchInput=off
  SR : Inport  Port=5  LatchInput=off
  Memory : Memory  X0=0  InheritSampleTime=off
      settings: RTWStateStorageClass=Auto
  Memory1 : Memory  X0=0  InheritSampleTime=off
      settings: RTWStateStorageClass=Auto
  MinMax : MinMax  Function=min  Inputs=2
  TR Look-Up Table TR=Tout/Tin : Lookup  InputValues=htc_sr  OutputValues=htc_tr
  T_max : Subsystem
      settings: RTWFcnNameOpts=Auto  RTWFileNameOpts=Auto
  Tin*TR= Tout,req : Product  Inputs=2  Multiplication=Element-wise(.*)  SaturateOnIntegerOverflow=on
  engine speed estimator : Subsystem
      settings: RTWFcnNameOpts=Auto  RTWFileNameOpts=Auto
  "shifting, override zero Trequest" : Switch  Threshold=eps
  T req : Outport  Port=1
  wires:
  Tin*TR= Tout,req/1 -> Memory/1
  TR/1 -> Tin*TR= Tout,req/2
  Req'd  input trq/1 -> Tin*TR= Tout,req/1
  Memory/1 -> "shifting, override zero Trequest"/1
  T_max/1(T_max max gain from htc) -> MinMax/2
  "shifting, override zero Trequest"/1 -> MinMax/1
  TR Look-Up Table TR=Tout/Tin/1 -> T_max/2(TR)
  MinMax/1 -> T req/1
  engine speed estimator/1(Out1) -> T_max/1(w_APU)
  Memory1/1 -> TR Look-Up Table TR=Tout/Tin/1
  SR/1 -> Memory1/1
  htc_spd_in_a/1 -> engine speed estimator/1(htc_spd_in_a)
  Req'd output trq/1 -> "shifting, override zero Trequest"/3
  [shifting] -> "shifting, override zero Trequest"/2

== system lib_transmission/hydraulic torque converter for  parallel hybrid <htc>/TR ==
  SR : Inport  Port=1  LatchInput=off
  coasting : Inport  Port=2  LatchInput=off
  1/SR*TR  for coast : Fcn  Expr=1/u
  Constant3 : Constant  Value=1
  Logical Operator : Logic  Operator=NOT  Inputs=1
  Logical Operator1 : Logic  Operator=NOT  Inputs=1
  TR Look-Up Table TR=Tout/Tin : Lookup  InputValues=htc_sr  OutputValues=htc_tr
  TR Look-Up Table TR=Tout/Tin coast : Lookup  InputValues=htc_sr_coast  OutputValues=htc_tr_coast
  To Workspace11 : ToWorkspace  VariableName=htc_efficiency  SampleTime=-1  SaveFormat=Array
  effic=SR*TR : Product  Inputs=**  Multiplication=Element-wise(.*)  SaturateOnIntegerOverflow=on
  if coasting : Switch  Threshold=eps
  if coasting1 : Switch  Threshold=eps
  "locked up, then TR=1" : Switch  Threshold=eps
  min,max : Saturate  UpperLimit=htc_max_coast_tr  LowerLimit=htc_min_coast_tr  LinearizeAsGain=on
  TR : Outport  Port=1  InitialOutput=0
  wires:
  if coasting1/1 -> To Workspace11/1
  1/SR*TR  for coast/1 -> if coasting1/3
  effic=SR*TR/1 -> 1/SR*TR  for coast/1, if coasting1/1
  Logical Operator1/1 -> if coasting1/2, if coasting/2
  if coasting/1 -> effic=SR*TR/2, TR/1
  coasting/1 -> Logical Operator1/1
  SR/1 -> effic=SR*TR/1, TR Look-Up Table TR=Tout/Tin/1, TR Look-Up Table TR=Tout/Tin coast/1
  min,max/1 -> if coasting/3
  TR Look-Up Table TR=Tout/Tin coast/1 -> min,max/1
  "locked up, then TR=1"/1 -> if coasting/1
  Logical Operator/1 -> "locked up, then TR=1"/2
  [locked_up] -> Logical Operator/1
  Constant3/1 -> "locked up, then TR=1"/3
  TR Look-Up Table TR=Tout/Tin/1 -> "locked up, then TR=1"/1

== system lib_transmission/hydraulic torque converter for  parallel hybrid <htc>/effect of inertia (Nm) ==
  note: This block computes the torque required to overcome the inertia of the
      | turbine (plus 1/2 fluid in htc).
  turbine/output speed (rad/s) : Inport  Port=1  LatchInput=off
  Constant : Constant  Value=htc_inertia
  Product : Product  Inputs=2  Multiplication=Element-wise(.*)  SaturateOnIntegerOverflow=on
  d/dt : Derivative
  inertia torque (Nm) : Outport  Port=1  InitialOutput=0
  wires:
  Product/1 -> inertia torque (Nm)/1
  Constant/1 -> Product/2
  turbine/output speed (rad/s)/1 -> d/dt/1
  d/dt/1 -> Product/1

== system lib_transmission/torque coupler <tc>/Block NOTES ==
  note: This block models a chain- or belt-driven torque coupler, with three gears:  one each
      | for the motor, main input (the engine or gearbox), and main output (to the gearbox
      | or final drive).  It includes losses in the chain or belt, but leaves inertia effects to be
      | considered in the appropriate component.
      |
      | The entire torque required out of the torque coupler (plus losses) is required from the
      | engine.  The engine provides only as much torque as its engine controller (see the
      | <vc> block) allows.  Any remaining unmet torque request is submitted to the motor,
      | which meets the request to the best of its ability.
      |
      | The torque converter output speed is limited by the maximum speeds of both the
      | motor and the engine.
      |
      | The loss torque is zero when the gears are not turning, and is applied at the output
      |  gear.
      |
      | The gears connecting the main input and main output to the torque converter's belt
      | or chain are assumed to be of the same size, so that main input speed = main output
  note: speed, while the motor's speed may be different.  The ratio of motor speed to main
      | output speed is stored in the variable tc_mc_to_fc_spd_ratio.

== system lib_transmission/torque coupler <tc>/help ==

== system lib_transmission/torque coupler <tc>/loss (Nm) ==
  note: The loss torque is zero when the gears are not turning,
      | and is applied at the torque coupler's output gear.
  tc output speed (rad/s) : Inport  Port=1  LatchInput=off
  Constant : Constant  Orientation=up  Value=0
  Switch : Switch  Threshold=eps
  torque coupler loss torque (Nm) : Constant  Value=tc_loss
  drag torque (Nm) : Outport  Port=1  InitialOutput=0
  wires:
  Constant/1 -> Switch/3
  tc output speed (rad/s)/1 -> Switch/2
  Switch/1 -> drag torque (Nm)/1
  torque coupler loss torque (Nm)/1 -> Switch/1

== system lib_transmission/torque coupler <tc> DIRECT SPLIT/Block NOTES ==
  note: This block generically models a chain- or belt-driven torque coupler, with three gears:  one each
      | for the motor, main input (the engine or gearbox), and main output (to the gearbox
      | or final drive).  It includes losses in the chain or belt, but leaves inertia effects to be
      | considered in the appropriate component.
      |
      | The entire torque required out of the torque coupler (plus losses) is sent to the control
      | strategy. The control strategy <CS> then decides how much the electric motor
      | and the ICE must supply. It then sends the EM and ICE separate requests. The 2 sources
      | then send their achieved torque signals to the Torque Coupler, where they are added
      | and sent to the block immediately before this.
      |
      | The torque coupler output speed is limited by the maximum speeds of both the
      | motor and the engine. The loss torque is zero when the gears are not
      | turning, and is applied at the output gear.
      |
      | The gears connecting the main input and main output to the torque converter's belt
      | or chain are assumed to be of the same size, so that main input speed = main output
      | speed, while the motor's speed may be different.  The ratio of motor speed to main
      | output speed is stored in the variable tc_mc_to_fc_spd_ratio.
      |
      | NOTE: This block is modeled after the HONDA Insight. It represents a hypothetical Torque
      | Coupler, since in the Insight, the EM and ICE are on the same shaft. Change the
      | values of the ratio and inertia if modeling another torque coupler.

== system lib_transmission/torque coupler <tc> DIRECT SPLIT/help ==

== system lib_transmission/torque coupler <tc> DIRECT SPLIT/loss (Nm) ==
  note: The loss torque is zero when the gears are not turning,
      | and is applied at the torque coupler's output gear.
      |
      | FOR THE INSIGHT, tc_loss==0
  tc output speed (rad/s) : Inport  Port=1  LatchInput=off
  Constant : Constant  Orientation=up  Value=0
  Switch : Switch  Threshold=eps
  torque coupler loss torque (Nm) : Constant  Value=tc_loss
  drag torque (Nm) : Outport  Port=1  InitialOutput=0
  wires:
  torque coupler loss torque (Nm)/1 -> Switch/1
  Switch/1 -> drag torque (Nm)/1
  tc output speed (rad/s)/1 -> Switch/2
  Constant/1 -> Switch/3
